simulink model "PI_SMC_Comparison"  (R2024a)
settings: Solver=ode1  StartTime=0.0  StopTime=1  RelTol=1e-3
values from neighbouring files (symbols this model uses):
  C = 100e-6    (= 0.0001)    [converter_parameter.m]
  V_fc = 14.4    [converter_parameter.m]
undefined symbols (not defined in the file or in its folder): plecs, sigbuilder_block
libraries: eePwmGenerator x4
settings Model: Creator=qaromose  LastModifiedBy=QUDUS
settings DebuggingCC: UnconnectedInputMsg=warning  UnconnectedOutputMsg=warning  UnconnectedLineMsg=warning
settings ModelReferenceCC: EnableRefExpFcnMdlSchedulingChecks=on
settings RTWCC: GPUComputeCapability=3.5  DLArmComputeVersion=19.05

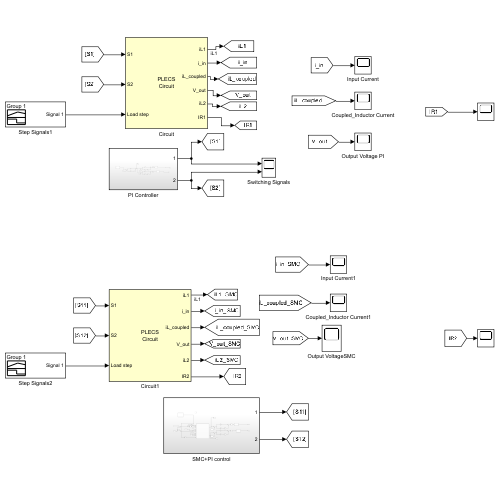
[thumbnail: Simulink's stored preview of the top-level diagram]
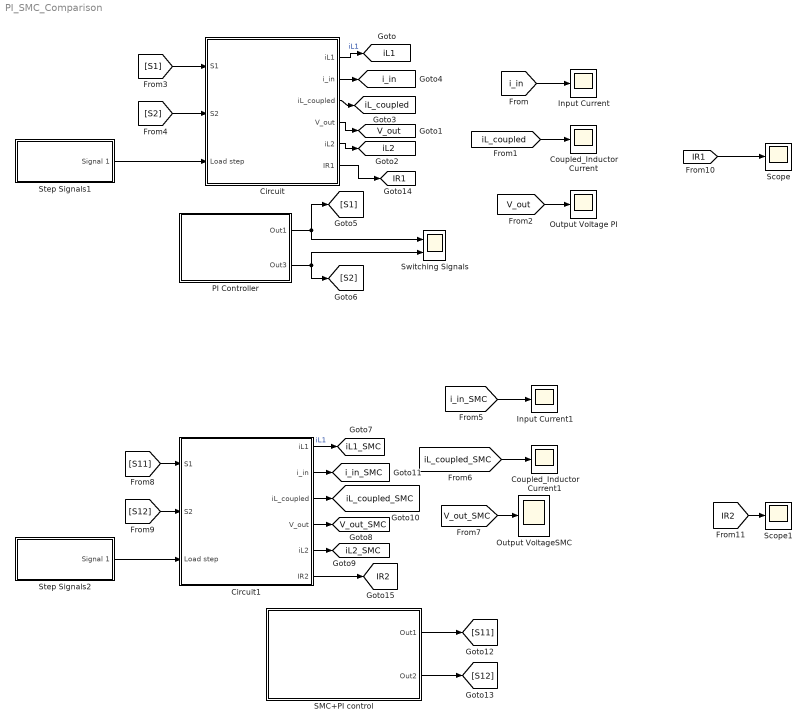
== system PI_SMC_Comparison ==
  Circuit : Subsystem  LoadFcn=plecs('sl', 200);  InitFcn=plecs('sl', 214);  StartFcn=plecs('sl', 208);  StopFcn=plecs('sl', 209);  mask(PlecsCircuit){PLECSData=<binary blob, 4280 chars, not shown>}
      mask prompts: PLECSData "PLECS Data (Do not delete or modify!)"
      mask init:
      | % PLACE CUSTOM INITIALIZATIONS ABOVE
      | % DO NOT REMOVE
      | plecs('sl', 215);
      | % DO NOT REMOVE
      settings: CopyFcn=plecs('sl', 203);  DeleteFcn=plecs('sl', 205);  UndoDeleteFcn=plecs('sl', 206);  PreSaveFcn=plecs('sl', 211);  PostSaveFcn=plecs('sl', 201);  NameChangeFcn=plecs('sl', 210);  DestroyFcn=plecs('sl', 207);  PreCopyFcn=plecs('sl', 216);  OpenFcn=plecs('sl', 202);  ErrorFcn=plerrorfcn
      mask Help: eval('plecs(''help'', ''qthelp:///creatingacircuit.html'')')
      mask Display: disp('PLECS\nCircuit')
  Circuit1 : Subsystem  LoadFcn=plecs('sl', 200);  InitFcn=plecs('sl', 214);  StartFcn=plecs('sl', 208);  StopFcn=plecs('sl', 209);  mask(PlecsCircuit){PLECSData=<binary blob, 4624 chars, not shown>}
      mask prompts: PLECSData "PLECS Data (Do not delete or modify!)"
      mask init:
      | % PLACE CUSTOM INITIALIZATIONS ABOVE
      | % DO NOT REMOVE
      | plecs('sl', 215);
      | % DO NOT REMOVE
      settings: CopyFcn=plecs('sl', 203);  DeleteFcn=plecs('sl', 205);  UndoDeleteFcn=plecs('sl', 206);  PreSaveFcn=plecs('sl', 211);  PostSaveFcn=plecs('sl', 201);  NameChangeFcn=plecs('sl', 210);  DestroyFcn=plecs('sl', 207);  PreCopyFcn=plecs('sl', 216);  OpenFcn=plecs('sl', 202);  ErrorFcn=plerrorfcn
      mask Help: eval('plecs(''help'', ''qthelp:///creatingacircuit.html'')')
      mask Display: disp('PLECS\nCircuit')
  Coupled_Inductor Current : Scope
  Coupled_Inductor Current1 : Scope
  Input Current : Scope
  Input Current1 : Scope
  Output Voltage PI : Scope
  Output VoltageSMC : Scope
  PI Controller : Subsystem
  SMC+PI control : Subsystem
  Scope : Scope
  Scope1 : Scope
  Step Signals1 : Subsystem  Tag=STV Subsys  LoadFcn=sigbuilder_block('load');  StartFcn=sigbuilder_block('start');  StopFcn=sigbuilder_block('stop');  ClipboardFcn=sigbuilder_block('clipboard');  mask(Sigbuilder block){tuvar=[0:10]}
      mask help: Simulink:masks:SigbuilderBlock_MD
      mask init:
      | if ~strcmp(get_param(bdroot(gcbh),'SimulationStatus'),'stopped') tuvar = sigbuilder_block('maskInit'); end
      settings: CopyFcn=sigbuilder_block('copy');  DeleteFcn=sigbuilder_block('delete');  ModelCloseFcn=sigbuilder_block('modelClose');  PreSaveFcn=sigbuilder_block('preSave');  PauseFcn=sigbuilder_block('pause');  ContinueFcn=sigbuilder_block('continue');  NameChangeFcn=sigbuilder_block('namechange');  OpenFcn=sigbuilder_block('open',[5.4 5.4 1141.2 580.8 ]);  CloseFcn=sigbuilder_block('close');
      mask Display: plot(0, 0, 100, 100,[2, 2, 32, 32, 2], [68, 8, 8, 68, 68],[32, 2], [38, 38], [32, 19, 2],[53, 60, 44], [32, 17, 17, 2],[16, 16, 31, 31]);txt = getActiveGroup(gcbh);text(2, 100, txt,'verticalAlignment', 'top');
  Step Signals2 : Subsystem  Tag=STV Subsys  LoadFcn=sigbuilder_block('load');  StartFcn=sigbuilder_block('start');  StopFcn=sigbuilder_block('stop');  ClipboardFcn=sigbuilder_block('clipboard');  mask(Sigbuilder block){tuvar=[0:10]}
      mask help: Simulink:masks:SigbuilderBlock_MD
      mask init:
      | if ~strcmp(get_param(bdroot(gcbh),'SimulationStatus'),'stopped') tuvar = sigbuilder_block('maskInit'); end
      settings: CopyFcn=sigbuilder_block('copy');  DeleteFcn=sigbuilder_block('delete');  ModelCloseFcn=sigbuilder_block('modelClose');  PreSaveFcn=sigbuilder_block('preSave');  PauseFcn=sigbuilder_block('pause');  ContinueFcn=sigbuilder_block('continue');  NameChangeFcn=sigbuilder_block('namechange');  OpenFcn=sigbuilder_block('open',[5.4 5.4 1141.2 580.8 ]);  CloseFcn=sigbuilder_block('close');
      mask Display: plot(0, 0, 100, 100,[2, 2, 32, 32, 2], [68, 8, 8, 68, 68],[32, 2], [38, 38], [32, 19, 2],[53, 60, 44], [32, 17, 17, 2],[16, 16, 31, 31]);txt = getActiveGroup(gcbh);text(2, 100, txt,'verticalAlignment', 'top');
  Switching Signals : Scope  NumInputPorts=2
  tag scope: IR1=global, IR2=global, V_out=global, V_out_SMC=global, iL1=global, iL1_SMC=global, iL2=global, iL2_SMC=global, iL_coupled=global, iL_coupled_SMC=global, i_in=global, i_in_SMC=global
  wires:
  [i_in] -> Input Current/1
  PI Controller/2(Out3) -> Switching Signals/2, [S2]
  [V_out] -> Output Voltage PI/1
  [S1] -> Circuit/1(S1)
  PI Controller/1(Out1) -> [S1], Switching Signals/1
  [iL_coupled] -> Coupled_Inductor Current/1
  Circuit/1(iL1) -> [iL1]  "iL1"
  Circuit/5(iL2) -> [iL2]
  Circuit/2(i_in) -> [i_in]
  Circuit/3(iL_coupled) -> [iL_coupled]
  Circuit/4(V_out) -> [V_out]
  [S2] -> Circuit/2(S2)
  Circuit1/3(iL_coupled) -> [iL_coupled_SMC]
  SMC+PI control/2(Out2) -> [S12]
  [V_out_SMC] -> Output VoltageSMC/1
  Circuit1/5(iL2) -> [iL2_SMC]
  [S11] -> Circuit1/1(S1)
  [S12] -> Circuit1/2(S2)
  Circuit1/2(i_in) -> [i_in_SMC]
  [iL_coupled_SMC] -> Coupled_Inductor Current1/1
  Circuit1/1(iL1) -> [iL1_SMC]  "iL1"
  SMC+PI control/1(Out1) -> [S11]
  Circuit1/4(V_out) -> [V_out_SMC]
  [i_in_SMC] -> Input Current1/1
  Circuit/6(IR1) -> [IR1]
  [IR1] -> Scope/1
  Circuit1/6(IR2) -> [IR2]
  [IR2] -> Scope1/1
  Step Signals1/1(Signal 1) -> Circuit/3(Load step)
  Step Signals2/1(Signal 1) -> Circuit1/3(Load step)

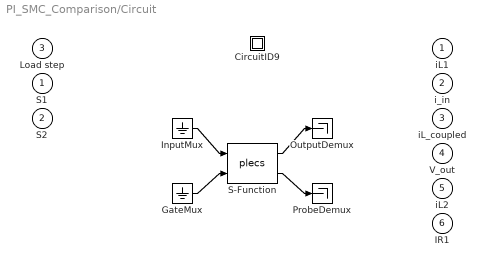
== system PI_SMC_Comparison/Circuit ==
  S1 : Inport  PortDimensions=1
  S2 : Inport  Port=2  PortDimensions=1
  Load step : Inport  Port=3  PortDimensions=1
  " CircuitID9 " : Subsystem
  " GateMux " : Ground
  " InputMux " : Ground
  " OutputDemux " : Terminator
  " ProbeDemux " : Terminator
  " S-Function " : S-Function  FunctionName=plecs  SFunctionDeploymentMode=off  EnableBusSupport=off
  iL1 : Outport  PortDimensions=1
  i_in : Outport  Port=2  PortDimensions=1
  iL_coupled : Outport  Port=3  PortDimensions=2
  V_out : Outport  Port=4  PortDimensions=1
  iL2 : Outport  Port=5  PortDimensions=1
  IR1 : Outport  Port=6  PortDimensions=1
  wires:
  " InputMux "/1 -> " S-Function "/1
  " GateMux "/1 -> " S-Function "/2
  " S-Function "/1 -> " OutputDemux "/1
  " S-Function "/2 -> " ProbeDemux "/1

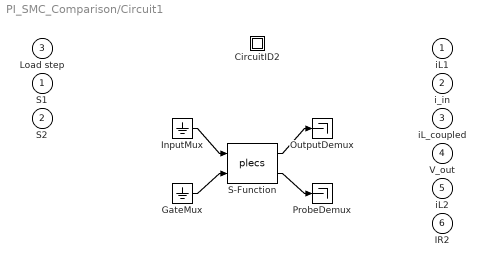
== system PI_SMC_Comparison/Circuit1 ==
  S1 : Inport  PortDimensions=1
  S2 : Inport  Port=2  PortDimensions=1
  Load step : Inport  Port=3  PortDimensions=1
  " CircuitID2 " : Subsystem
  " GateMux " : Ground
  " InputMux " : Ground
  " OutputDemux " : Terminator
  " ProbeDemux " : Terminator
  " S-Function " : S-Function  FunctionName=plecs  SFunctionDeploymentMode=off  EnableBusSupport=off
  iL1 : Outport  PortDimensions=1
  i_in : Outport  Port=2  PortDimensions=1
  iL_coupled : Outport  Port=3  PortDimensions=2
  V_out : Outport  Port=4  PortDimensions=1
  iL2 : Outport  Port=5  PortDimensions=1
  IR2 : Outport  Port=6  PortDimensions=1
  wires:
  " InputMux "/1 -> " S-Function "/1
  " GateMux "/1 -> " S-Function "/2
  " S-Function "/1 -> " OutputDemux "/1
  " S-Function "/2 -> " ProbeDemux "/1

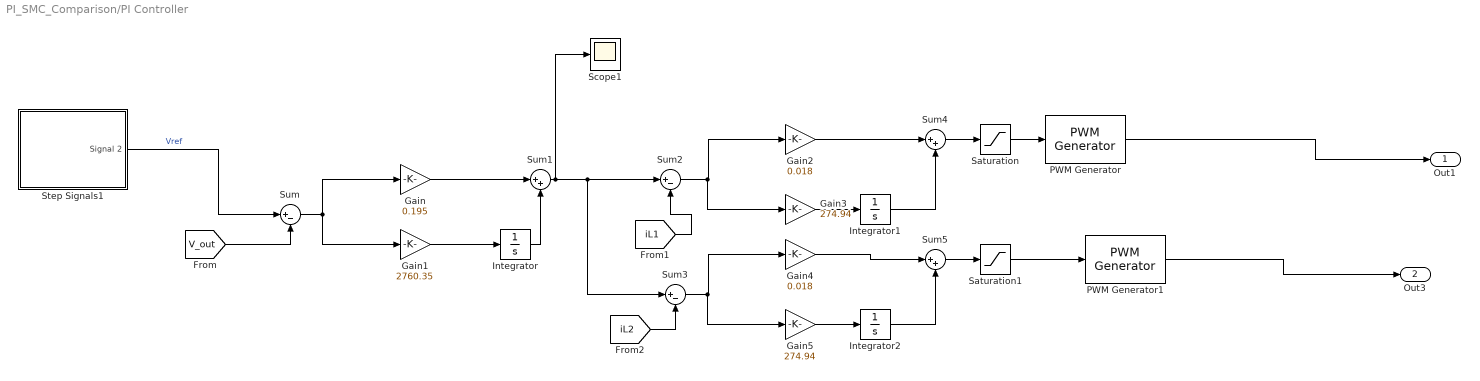
== system PI_SMC_Comparison/PI Controller ==
  Gain : Gain  Gain=0.195
  Gain1 : Gain  Gain=2760.35
  Gain2 : Gain  Gain=0.018
  Gain3 : Gain  Gain=274.94
  Gain4 : Gain  Gain=0.018
  Gain5 : Gain  Gain=274.94
  Integrator : Integrator
  Integrator1 : Integrator
  Integrator2 : Integrator
  PWM Generator : eePwmGenerator/PWM Generator  CarrCount=Up  Tper=2e-5  Tdelay=0  Ts=0
  PWM Generator1 : eePwmGenerator/PWM Generator  CarrCount=Up  Tper=2e-5  Tdelay=1e-5  Ts=0
  Saturation : Saturate  UpperLimit=0.9  LowerLimit=0.1
  Saturation1 : Saturate  UpperLimit=0.9  LowerLimit=0.1
  Scope1 : Scope
  Step Signals1 : Subsystem  Tag=STV Subsys  LoadFcn=sigbuilder_block('load');  StartFcn=sigbuilder_block('start');  StopFcn=sigbuilder_block('stop');  ClipboardFcn=sigbuilder_block('clipboard');  mask(Sigbuilder block){tuvar=[0:10]}
      mask help: Simulink:masks:SigbuilderBlock_MD
      mask init:
      | if ~strcmp(get_param(bdroot(gcbh),'SimulationStatus'),'stopped') tuvar = sigbuilder_block('maskInit'); end
      settings: CopyFcn=sigbuilder_block('copy');  DeleteFcn=sigbuilder_block('delete');  ModelCloseFcn=sigbuilder_block('modelClose');  PreSaveFcn=sigbuilder_block('preSave');  PauseFcn=sigbuilder_block('pause');  ContinueFcn=sigbuilder_block('continue');  NameChangeFcn=sigbuilder_block('namechange');  OpenFcn=sigbuilder_block('open',[5.4 5.4 1141.2 580.8 ]);  CloseFcn=sigbuilder_block('close');
      mask Display: plot(0, 0, 100, 100,[2, 2, 32, 32, 2], [68, 8, 8, 68, 68],[32, 2], [38, 38], [32, 19, 2],[53, 60, 44], [32, 17, 17, 2],[16, 16, 31, 31]);txt = getActiveGroup(gcbh);text(2, 100, txt,'verticalAlignment', 'top');
  Sum : Sum  Inputs=|+-
  Sum1 : Sum  Inputs=|++
  Sum2 : Sum  Inputs=|+-
  Sum3 : Sum  Inputs=|+-
  Sum4 : Sum  Inputs=|++
  Sum5 : Sum  Inputs=|++
  Out1 : Outport
  Out3 : Outport  Port=2
  wires:
  [V_out] -> Sum/2
  Gain5/1 -> Integrator2/1
  Sum1/1 -> Sum3/1, Sum2/1, Scope1/1
  Gain4/1 -> Sum5/1
  Gain2/1 -> Sum4/1
  Sum3/1 -> Gain5/1, Gain4/1
  Integrator1/1 -> Sum4/2
  Integrator2/1 -> Sum5/2
  [iL1] -> Sum2/2
  Gain1/1 -> Integrator/1
  [iL2] -> Sum3/2
  Sum/1 -> Gain1/1, Gain/1
  Sum2/1 -> Gain3/1, Gain2/1
  Integrator/1 -> Sum1/2
  Saturation/1 -> PWM Generator/1
  Gain/1 -> Sum1/1
  Gain3/1 -> Integrator1/1
  Sum5/1 -> Saturation1/1
  Sum4/1 -> Saturation/1
  Saturation1/1 -> PWM Generator1/1
  PWM Generator/1 -> Out1/1
  Step Signals1/1(Signal 2) -> Sum/1  "Vref"
  PWM Generator1/1 -> Out3/1

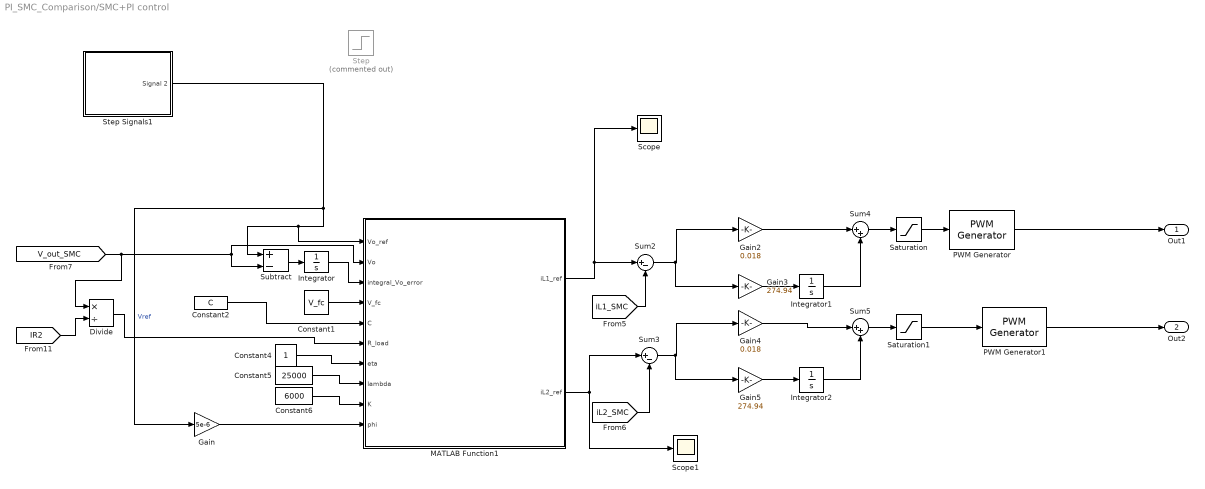
== system PI_SMC_Comparison/SMC+PI control ==
  Constant1 : Constant  Value=V_fc
  Constant2 : Constant  Value=C
  Constant4 : Constant
  Constant5 : Constant  Value=25000
  Constant6 : Constant  Value=6000
  Divide : Product  Inputs=*/  RndMeth=Zero  SaturateOnIntegerOverflow=on
  Gain : Gain  Gain=5e-6
  Gain2 : Gain  Gain=0.018
  Gain3 : Gain  Gain=274.94
  Gain4 : Gain  Gain=0.018
  Gain5 : Gain  Gain=274.94
  Integrator : Integrator
  Integrator1 : Integrator
  Integrator2 : Integrator
  MATLAB Function1 : MATLAB Function  TreatAsAtomicUnit=on
  PWM Generator : eePwmGenerator/PWM Generator  CarrCount=Up  Tper=2e-5  Tdelay=0  Ts=0
  PWM Generator1 : eePwmGenerator/PWM Generator  CarrCount=Up  Tper=2e-5  Tdelay=1e-5  Ts=0
  Saturation : Saturate  UpperLimit=0.97  LowerLimit=0.1
  Saturation1 : Saturate  UpperLimit=0.97  LowerLimit=0.1
  Scope : Scope
  Scope1 : Scope
  Step : Step  Commented=on  Time=0.2  Before=48  After=40  SampleTime=0
  Step Signals1 : Subsystem  Tag=STV Subsys  LoadFcn=sigbuilder_block('load');  StartFcn=sigbuilder_block('start');  StopFcn=sigbuilder_block('stop');  ClipboardFcn=sigbuilder_block('clipboard');  mask(Sigbuilder block){tuvar=[0:10]}
      mask help: Simulink:masks:SigbuilderBlock_MD
      mask init:
      | if ~strcmp(get_param(bdroot(gcbh),'SimulationStatus'),'stopped') tuvar = sigbuilder_block('maskInit'); end
      settings: CopyFcn=sigbuilder_block('copy');  DeleteFcn=sigbuilder_block('delete');  ModelCloseFcn=sigbuilder_block('modelClose');  PreSaveFcn=sigbuilder_block('preSave');  PauseFcn=sigbuilder_block('pause');  ContinueFcn=sigbuilder_block('continue');  NameChangeFcn=sigbuilder_block('namechange');  OpenFcn=sigbuilder_block('open',[5.4 5.4 1141.2 580.8 ]);  CloseFcn=sigbuilder_block('close');
      mask Display: plot(0, 0, 100, 100,[2, 2, 32, 32, 2], [68, 8, 8, 68, 68],[32, 2], [38, 38], [32, 19, 2],[53, 60, 44], [32, 17, 17, 2],[16, 16, 31, 31]);txt = getActiveGroup(gcbh);text(2, 100, txt,'verticalAlignment', 'top');
  Subtract : Sum  Inputs=+-
  Sum2 : Sum  Inputs=|+-
  Sum3 : Sum  Inputs=|+-
  Sum4 : Sum  Inputs=|++
  Sum5 : Sum  Inputs=|++
  Out1 : Outport
  Out2 : Outport  Port=2
  wires:
  Sum2/1 -> Gain3/1, Gain2/1
  [V_out_SMC] -> Divide/1, MATLAB Function1/2(Vo), Subtract/2
  Saturation/1 -> PWM Generator/1
  [iL1_SMC] -> Sum2/2
  Subtract/1 -> Integrator/1
  Sum3/1 -> Gain5/1, Gain4/1
  MATLAB Function1/1(iL1_ref) -> Scope/1, Sum2/1
  MATLAB Function1/2(iL2_ref) -> Sum3/1, Scope1/1
  Gain4/1 -> Sum5/1
  Sum4/1 -> Saturation/1
  Gain5/1 -> Integrator2/1
  Integrator2/1 -> Sum5/2
  Gain3/1 -> Integrator1/1
  Integrator1/1 -> Sum4/2
  Integrator/1 -> MATLAB Function1/3(integral_Vo_error)
  Gain2/1 -> Sum4/1
  Saturation1/1 -> PWM Generator1/1
  Sum5/1 -> Saturation1/1
  [iL2_SMC] -> Sum3/2
  Constant2/1 -> MATLAB Function1/5(C)
  Divide/1 -> MATLAB Function1/6(R_load)
  Constant4/1 -> MATLAB Function1/7(eta)
  Constant5/1 -> MATLAB Function1/8(lambda)
  Constant6/1 -> MATLAB Function1/9(K)
  Gain/1 -> MATLAB Function1/10(phi)
  Constant1/1 -> MATLAB Function1/4(V_fc)
  Step Signals1/1(Signal 2) -> Gain/1, Subtract/1, MATLAB Function1/1(Vo_ref)  "Vref"
  [IR2] -> Divide/2
  PWM Generator1/1 -> Out2/1
  PWM Generator/1 -> Out1/1

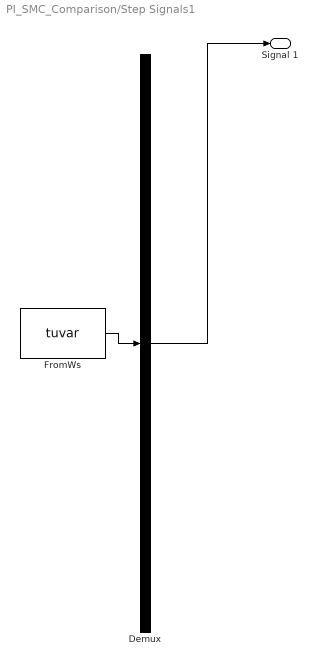
== system PI_SMC_Comparison/Step Signals1 ==
  Demux : Demux  Tag=STV Demux  Outputs=1
      settings: DisplayOption=none
  FromWs : FromWorkspace  Tag=STV FromWs  VariableName=tuvar
      SigBuilderData=|
      | common.afterFinalStr = 'Extrapolate'
      | common.sampleTime = 0
      | dataSet.timeRange = [0 35]
      | dataSet.name = 'Group 1'
      | sbobj.Groups.Name = 'Group 1'
      | sbobj.Groups.Signals.Name = 'Signal 1'
      | sbobj.Groups.Signals.XData = [0 0.101 0.101 0.301 0.301 35]
      | sbobj.Groups.Signals.YData = [0 0 5 5 0 0]
      | sbobj.Groups.TimeRange = [0 35]
  Signal 1 : Outport  Tag=STV Outport
  wires:
  FromWs/1 -> Demux/1
  Demux/1 -> Signal 1/1

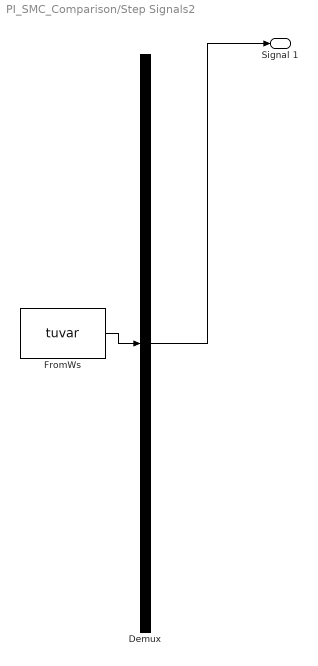
== system PI_SMC_Comparison/Step Signals2 ==
  Demux : Demux  Tag=STV Demux  Outputs=1
      settings: DisplayOption=none
  FromWs : FromWorkspace  Tag=STV FromWs  VariableName=tuvar
      SigBuilderData=|
      | common.afterFinalStr = 'Extrapolate'
      | common.sampleTime = 0
      | dataSet.timeRange = [0 35]
      | dataSet.name = 'Group 1'
      | sbobj.Groups.Name = 'Group 1'
      | sbobj.Groups.Signals.Name = 'Signal 1'
      | sbobj.Groups.Signals.XData = [0 0.101 0.101 0.301 0.301 35]
      | sbobj.Groups.Signals.YData = [0 0 5 5 0 0]
      | sbobj.Groups.TimeRange = [0 35]
  Signal 1 : Outport  Tag=STV Outport
  wires:
  FromWs/1 -> Demux/1
  Demux/1 -> Signal 1/1

== system PI_SMC_Comparison/Circuit/ CircuitID9  ==

== system PI_SMC_Comparison/Circuit1/ CircuitID2  ==

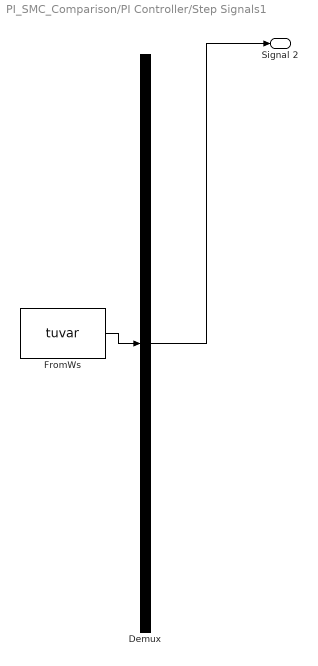
== system PI_SMC_Comparison/PI Controller/Step Signals1 ==
  Demux : Demux  Tag=STV Demux  Outputs=1
      settings: DisplayOption=none
  FromWs : FromWorkspace  Tag=STV FromWs  VariableName=tuvar
      SigBuilderData=|
      | common.afterFinalStr = 'Extrapolate'
      | common.sampleTime = 0
      | dataSet.timeRange = [0 35]
      | dataSet.name = 'Group 1'
      | sbobj.Groups.Name = 'Group 1'
      | sbobj.Groups.Signals.Name = 'Signal 2'
      | sbobj.Groups.Signals.XData = [0 0.01 0.2 0.2 0.4 0.4 0.6 0.6 0.801 0.801 1.01 1.01 20.001 20.001 25 25 35]
      | sbobj.Groups.Signals.YData = [60 60 60 48 48 40 40 30 30 48 47.5 0 84 122 122 98.5 97]
      | sbobj.Groups.TimeRange = [0 35]
  Signal 2 : Outport  Tag=STV Outport
  wires:
  Demux/1 -> Signal 2/1
  FromWs/1 -> Demux/1

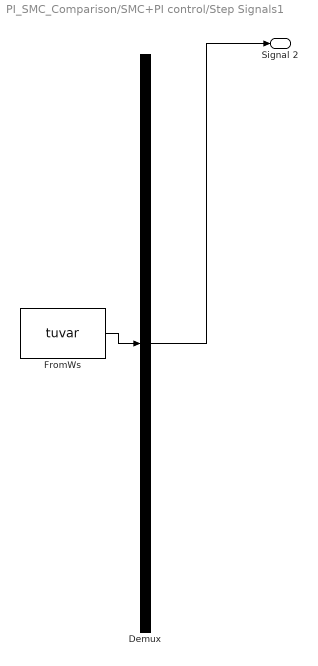
== system PI_SMC_Comparison/SMC+PI control/Step Signals1 ==
  Demux : Demux  Tag=STV Demux  Outputs=1
      settings: DisplayOption=none
  FromWs : FromWorkspace  Tag=STV FromWs  VariableName=tuvar
      SigBuilderData=|
      | common.afterFinalStr = 'Extrapolate'
      | common.sampleTime = 0
      | dataSet.timeRange = [0 35]
      | dataSet.name = 'Group 1'
      | sbobj.Groups.Name = 'Group 1'
      | sbobj.Groups.Signals.Name = 'Signal 2'
      | sbobj.Groups.Signals.XData = [0 0.01 0.2 0.2 0.4 0.4 0.6 0.6 0.801 0.801 1.01 1.01 20.001 20.001 25 25 35]
      | sbobj.Groups.Signals.YData = [60 60 60 48 48 40 40 30 30 48 47.5 0 84 122 122 98.5 97]
      | sbobj.Groups.TimeRange = [0 35]
  Signal 2 : Outport  Tag=STV Outport
  wires:
  Demux/1 -> Signal 2/1
  FromWs/1 -> Demux/1

== matlab function PI_SMC_Comparison/SMC+PI control/MATLAB Function1 ==
  data: Vo_ref input; Vo input; integral_Vo_error input; iL1_ref output; iL2_ref output; V_fc input; C input; R_load input; eta input; lambda input; K input; phi input
function [iL1_ref, iL2_ref] = Outer_SMC(Vo_ref, Vo, integral_Vo_error, V_fc, C, R_load, eta, lambda, K, phi)
    %% System Parameters (Optimized for ±0.5V Error)
%     V_fc = 14.4;          % Input voltage [V] (measured under load)
%     C = 100e-6;          % Output capacitance [F] 
%     R_load = 5;          % Load resistance [Ω] (48V/500W = 4.608Ω, adjust if needed)
%     eta = 0.97;          % desired efficiency (compensate for losses at higher Vo)
%     lambda = 25000;       % Aggressive integral gain (eliminate steady-state error)
%     K = 6000;             % High robustness gain (dominate uncertainties)
%     phi = 5e-6 * Vo_ref;% Adaptive boundary layer (0.5% of Vo_ref)
    
    %% Voltage error (Vo_ref - Vo)
    e_V = Vo_ref - Vo;
    
    %% Sliding surface
    S = e_V + lambda * integral_Vo_error;
    
    %% Adaptive boundary layer saturation
    if abs(S) <= phi
        sat_term = S / phi;   % Linear region
    else
        sat_term = sign(S);   % Reaching mode
    end
    
    %% Feedforward term (with efficiency compensation)
    iL_ref_eq = (Vo_ref^2) / (V_fc * R_load * eta);  % Critical adjustment
    
    %% Feedback term (scaled for precision)
    robustness_term = (C / V_fc) * (lambda * e_V + K * sat_term); 
    
    %% Total current reference (remove clamp or set hardware-safe limit)
    iL_ref_total = iL_ref_eq + robustness_term;
    % iL_ref_total = max(min(iL_ref_total, 100), 0);  % Example: 100A limit
    
    %% Split equally for 2-phase IBC
    iL1_ref = iL_ref_total / 2;  
    iL2_ref = iL_ref_total / 2;
end
